simulink library "HANcoder_Linux_Target"  (R2018b)
settings: Solver=ode45  StartTime=0.0  StopTime=10.0  RelTol=1e-3  EnableMultiTasking=on
settings Model: Creator=HANcoder  LastModifiedBy=rickg
settings Model: ModifiedHistory=|
  | la_obwlf -- Thu Sep 01 12:12:55 2016 -- Version 0.33
  | 
  | 
  | 
  | 
  | 
  | 
  | la_obwlf -- Thu Sep 01 09:23:34 2016 -- Version 0.33
  | changed the version in the Base Sample Time block
  | 
  | 
  | 
  | la_obwlf -- Tue Aug 30 15:48:17 2016 -- Version 0.33
settings DataIOCC: LimitDataPoints=on  SaveFormat=Array  SignalLoggingSaveFormat=ModelDataLogs
settings OptimizationCC: ExpressionDepthLimit=2147483647  LifeSpan=inf
settings DebuggingCC: UnderspecifiedInitializationDetection=Classic  MergeDetectMultiDrivingBlocksExec=none  SolverPrmCheckMsg=warning  FcnCallInpInsideContextMsg=warning  StateNameClashWarn=warning  SFUnexpectedBacktrackingDiag=warning  SFNoUnconditionalDefaultTransitionDiag=warning  SFExecutionAtInitializationDiag=none
settings HardwareCC: ProdBitPerPointer=32  ProdBitPerSizeT=32  ProdBitPerPtrDiffT=32  ProdLargestAtomicFloat=None  ProdIntDivRoundTo=Undefined  ProdEndianess=Unspecified  ProdWordSize=32  ProdHWDeviceType=32-bit Generic
settings ModelReferenceCC: PropagateSignalLabelsOutOfModel=off
settings SFSimCC: SimUseLocalCustomCode=off
settings RTWCC: RTWUseLocalCustomCode=off
settings CodeAppCC: StateflowObjectComments=on
settings GRTTargetCC: TargetLangStandard=C89/C90 (ANSI)  GeneratePreprocessorConditionals=Disable all  CombineOutputUpdateFcns=off  GRTInterface=on
settings ConfigComp: CovMetricSettings=dw  CovHtmlReporting=on  CovSaveCumulativeToWorkspaceVar=on  CovSaveSingleToWorkspaceVar=on  CovExternalEMLEnable=off  CovSFcnEnable=off

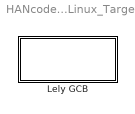
== system HANcoder_Linux_Target ==
  Lely GCB : Subsystem
      mask Display:
      | disp('Lely GCB')
      | patch([80 86 86],[8 14 2],[1 0 0]);patch([88 88 94],[14 2 8],[0 0 0.35]);

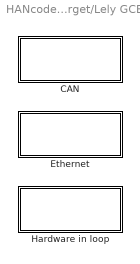
== system HANcoder_Linux_Target/Lely GCB ==
  CAN : Subsystem
      mask Display: fprintf('CAN');patch([85 91 91],[8 14 2],[1 0 0]);patch([93 93 99],[14 2 8],[0 0 0.35]);
  Ethernet : Subsystem
      mask Display: fprintf('Ethernet');patch([85 91 91],[8 14 2],[1 0 0]);patch([93 93 99],[14 2 8],[0 0 0.35]);
  Hardware in loop : Subsystem
      mask Display: fprintf('Hardware in the Loop');patch([85 91 91],[8 14 2],[1 0 0]);patch([93 93 99],[14 2 8],[0 0 0.35]);

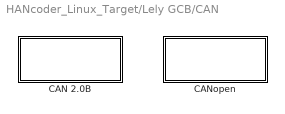
== system HANcoder_Linux_Target/Lely GCB/CAN ==
  CAN 2.0B : Subsystem
      mask Display: fprintf('CAN 2.0B');patch([85 91 91],[8 14 2],[1 0 0]);patch([93 93 99],[14 2 8],[0 0 0.35]);
  CANopen : Subsystem
      mask Display: fprintf('CANopen');patch([85 91 91],[8 14 2],[1 0 0]);patch([93 93 99],[14 2 8],[0 0 0.35]);

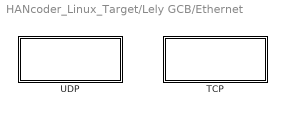
== system HANcoder_Linux_Target/Lely GCB/Ethernet ==
  TCP : Subsystem
      mask Display: fprintf('TCP');patch([85 91 91],[8 14 2],[1 0 0]);patch([93 93 99],[14 2 8],[0 0 0.35]);
  UDP : Subsystem
      mask Display: fprintf('UDP');patch([85 91 91],[8 14 2],[1 0 0]);patch([93 93 99],[14 2 8],[0 0 0.35]);

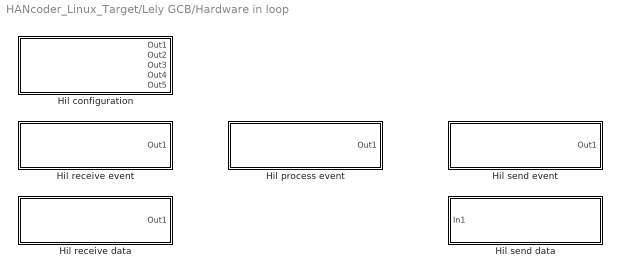
== system HANcoder_Linux_Target/Lely GCB/Hardware in loop ==
  Hil configuration : Subsystem  Tag=HANcoder_TARGET_STM32_Olimexino  mask{tsamp=1, hilSpeed=100, hilConf=HiL Master + 4 Slaves, hilTimeSlot=4, ip1=10, ip2=4, ip3=1, ip4=Automatically assigned by HiL}
      mask prompts: tsamp "Sample time"; hilSpeed "HiL cycle time (ms)"; hilConf "HiL configuration"; hilTimeSlot "Time slot to start"; ip1 "Adress 1"; ip2 "Adress 2"; ip3 "Adress 3"; ip4 "Adress 4"
      mask init:
      | configurationInfoString = sfcn_hil_mcb(hilConf,hilSpeed,hilTimeSlot,ip1,ip2,ip3)
      mask TypeOptions hilConf: HiL Master | HiL Master + 1 Slave | HiL Master + 2 Slaves | HiL Master + 3 Slaves | HiL Master + 4 Slaves
      mask TypeOptions hilTimeSlot: 4 | 5 | 6 | 7 | 8 | 9 | 10
      mask DialogControl Container4 Prompt: HiL parameters
      mask DialogControl Container3 Prompt: IO module IP range
      mask Display:
      | %%port_label('output', 1, 'Time slot');
      | %%port_label('output', 2, 'Sample counter');
      | %%port_label('output', 3, 'Samples lost');
      | %%port_label('output', 4, 'Plant model time');
      | fprintf('Hil Linux GCB\n Hil cycle speed: %d ms\n Setup: %s',hilSpeed,configurationInfoString);
      | patch([135 141 141],[8 14 2],[1 0 0]);patch([143 143 149],[14 2 8],[0 0 0.35]);
  Hil process event : Subsystem  Tag=HANcoder_TARGET_STM32_E407
      mask init:
      | sfcn_hil_process_irq_mcb();
      settings: MoveFcn=%%drawLogos
      mask Display: fprintf('Hil process\nInitiate process event');patch([135 141 141],[8 14 2],[1 0 0]);patch([143 143 149],[14 2 8],[0 0 0.35]);
  Hil receive data : Subsystem  Tag=HANcoder_TARGET_STM32_Olimexino  mask{ioModule=HiL Master, channel=1, datatype=int8}
      mask prompts: ioModule "Smart IO module"; channel "Signal channel"
      mask init:
      | [ioModuleinfoStr] = sfcn_hil_receive_data_mcb(ioModule, channel, datatype);
      mask TypeOptions ioModule: HiL Master | HiL Slave 1 | HiL Slave 2 | HiL Slave 3 | HiL Slave 4
      mask TypeOptions channel: 1 | 2 | 3 | 4 | 5 | 6 | 7 | 8 | 9 | 10 | 11 | 12 | 13 | 14 | 15 | 16 | 17 | 18 | 19 | 20
      mask TypeOptions datatype: int8 | uint8 | int16 | uint16 | int32 | uint32 | boolean
      mask Display: fprintf('Hil get data from\n%s\nChannel %d',ioModuleinfoStr, channel);patch([135 141 141],[8 14 2],[1 0 0]);patch([143 143 149],[14 2 8],[0 0 0.35]);
  Hil receive event : Subsystem  Tag=HANcoder_TARGET_STM32_E407
      mask init:
      | sfcn_hil_receive_irq_mcb();
      settings: MoveFcn=%%drawLogos
      mask Display: fprintf('Hil receive\nData received event');patch([135 141 141],[8 14 2],[1 0 0]);patch([143 143 149],[14 2 8],[0 0 0.35]);
  Hil send data : Subsystem  Tag=HANcoder_TARGET_STM32_Olimexino  mask{ioModule=HiL Master, channel=1, datatype=int8}
      mask prompts: ioModule "Smart IO module"; channel "Signal channel"
      mask init:
      | [ioModuleinfoStr] = sfcn_hil_send_data_mcb(ioModule, channel, datatype);
      mask TypeOptions ioModule: HiL Master | HiL Slave 1 | HiL Slave 2 | HiL Slave 3 | HiL Slave 4
      mask TypeOptions channel: 1 | 2 | 3 | 4 | 5 | 6 | 7 | 8 | 9 | 10 | 11 | 12 | 13 | 14 | 15 | 16 | 17 | 18 | 19 | 20
      mask TypeOptions datatype: int8 | uint8 | int16 | uint16 | int32 | uint32 | boolean
      mask Display: fprintf('Hil send data to\n%s\nChannel %d',ioModuleinfoStr, channel);patch([135 141 141],[8 14 2],[1 0 0]);patch([143 143 149],[14 2 8],[0 0 0.35]);
  Hil send event : Subsystem  Tag=HANcoder_TARGET_STM32_E407
      mask init:
      | sfcn_hil_send_irq_mcb();
      settings: MoveFcn=%%drawLogos
      mask Display: fprintf('Hil send\nInitiate send event');patch([135 141 141],[8 14 2],[1 0 0]);patch([143 143 149],[14 2 8],[0 0 0.35]);

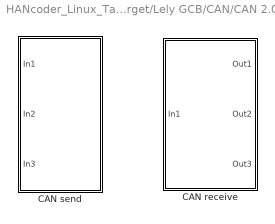
== system HANcoder_Linux_Target/Lely GCB/CAN/CAN 2.0B ==
  CAN receive : Subsystem  Tag=HANcoder_TARGET_STM32_Olimexino  mask(CAN receive){canBus=CAN 1, outputNumber=2, dataType=uint8, byteOrder=off, tsamp=1}
      mask prompts: canBus "CAN channel"; outputNumber "Output ports"; dataType "Output datatype"; byteOrder "Byte order: Checked = MSB first, unchecked = LSB first."; tsamp "Sample time"
      mask help:
      | Function
      | ==========
      | Receive the newest message from the specified CAN channel.
      |
      | Parameters
      | ==========
      | CAN channel:             The CAN channel to send the message on.
      | Output ports:             The amount of output ports
      | Output datatype:       The datatype of the output ports
      | Byte order:                 Select MSB or LSB first
      | Sample time:              -1 or divisible by base sample time [seconds]
      |
      | Input
      | ==========
      | Port 1:                       CAN ID(uint32) in hexadecimal ie: hex2dec('0a')
      |
      | Output
      | ==========
      | Port 1:                       Checks for new message(int8)
      | Port 2..9                     Message data
      mask init:
      | sfcn_can_receive_mcb(canBus, outputNumber, dataType, byteOrder)
      mask Help: web('sfcn_can_receive.html');
      mask TypeOptions canBus: CAN 1
      mask TypeOptions dataType: int8 | uint8 | int16 | uint16 | int32 | uint32 | boolean
      mask Display:
      | fprintf('Receive on\nCAN %x', canBus);
      | port_label('output', 1, 'new')
      | port_label('input', 1, 'ID');patch([75 81 81],[8 14 2],[1 0 0]);patch([83 83 89],[14 2 8],[0 0 0.35]);
  CAN send : Subsystem  Tag=HANcoder_TARGET_STM32_Olimexino  mask(CAN send){canBus=CAN0, frameType=Standard (11 bit), inputNumber=2, dataType=uint8, byteOrder=on, tsamp=0.5}
      mask prompts: canBus "CAN channel"; frameType "Identifier type"; inputNumber "Input ports"; dataType "Input datatype"; byteOrder "Byte order: Checked = MSB first, unchecked = LSB first."; tsamp "Sample time"
      mask help:
      | Function
      | ==========
      | Send a message on the CAN channel.
      |
      | Parameters
      | ==========
      | CAN channel:           The CAN channel to send the message on.
      | Identifier type:         normal or extended ID's
      | Input ports:              The amount of input ports
      | Input datatype:        The datatype of the input ports
      | Byte order:               Select MSB or LSB first
      | Sample time:            -1 or divisible by base sample time [seconds]
      |
      | Input
      | ==========
      | Port 1:                   CAN ID(uint32) in hexadecimal ie: hex2dec('0a')
      | Port 2..9                CAN message data
      mask init:
      | sfcn_can_send_mcb(canBus, frameType, inputNumber, dataType, byteOrder)
      mask Help: web('sfcn_can_send.html');
      mask TypeOptions canBus: CAN0 | CAN1
      mask TypeOptions frameType: Standard (11 bit) | Extended (29 bit)
      mask TypeOptions dataType: int8 | uint8 | int16 | uint16 | int32 | uint32 | boolean
      mask Display:
      | fprintf('Send on\nCAN%x', canBus-1);
      | port_label('input', 1, 'ID');patch([65 71 71],[8 14 2],[1 0 0]);patch([73 73 79],[14 2 8],[0 0 0.35]);

== system HANcoder_Linux_Target/Lely GCB/CAN/CANopen ==

== system HANcoder_Linux_Target/Lely GCB/Ethernet/TCP ==

== system HANcoder_Linux_Target/Lely GCB/Ethernet/UDP ==
  UDP Client Send : Subsystem  Tag=HANcoder_TARGET_STM32_Olimexino  mask(UDP Client Send){ip1=10, ip2=4, ip3=1, ip4=10, port=2000, inputNumber=1, dataType=int8, byteOrder=on, tsamp=-1}
      mask prompts: ip1 "IP address 1"; ip2 "IP address 2"; ip3 "IP address 3"; ip4 "IP address 4"; port "Port2"; inputNumber "Input ports"; dataType "Input datatype"; byteOrder "Byte order: Checked = MSB first, unchecked = LSB first."; tsamp "Sample time"
      mask help:
      | Function
      | ========
      | Sends a data packet to the UDP server with the specified IP address on
      | the specified port.
      |
      | Parameters
      | ==========
      | IP address 1:   First quad of the UDP server's IP address.
      | IP address 2:   Second quad of the UDP server's IP address.
      | IP address 3:   Third quad of the UDP server's IP address.
      | IP address 4:   Fourth quad of the UDP server's IP address.
      | Port:           Port to send the data packet on.
      | Input ports:    The amount of input ports.
      | Input datatype: The datatype of the input ports.
      | Byte order:     Select MSB or LSB first.
      | Sample time:    -1 or divisible by base sample time [seconds].
      |
      | Input
      | =====
      | Port 1..32      UDP packet data.
      mask init:
      | sfcn_udp_client_send_mcb(ip1,ip2,ip3,ip4,port,inputNumber,dataType,byteOrder);
      mask Help: web('sfcn_udp_client_send.html');
      mask TypeOptions inputNumber: 1 | 2 | 3 | 4 | 5 | 6 | 7 | 8 | 9 | 10 | 11 | 12 | 13 | 14 | 15 | 16 | 17 | 18 | 19 | 20 | 21 | 22 | 23 | 24 | 25 | 26 | 27 | 28 | 29 | 30 | 31 | 32
      mask TypeOptions dataType: int8 | uint8 | int16 | uint16 | int32 | uint32 | boolean
      mask Display:
      | fprintf('UDP Client Send');patch([125 131 131],[8 14 2],[1 0 0]);patch([133 133 139],[14 2 8],[0 0 0.35]);
      | %fprintf('UDP Client Send\n\nport: %d\nip: %d.%d.%d.%d', port, ip1, ip2, ip3, ip4);patch([125 131 131],[8 14 2],[1 0 0]);patch([133 133 139],[14 2 8],[0 0 0.35]);
  UDP Server Receive : Subsystem  Tag=HANcoder_TARGET_STM32_Olimexino  mask(UDP Server Receive){outputNumber=10, dataType=int8, byteOrder=on, startIdx=1, tsamp=-1}
      mask prompts: outputNumber "Output ports"; dataType "Output datatype"; byteOrder "Byte order: Checked = MSB first, unchecked = LSB first."; startIdx "Start index"; tsamp "Sample time"
      mask help:
      | Function
      | ========
      | Reads data from the UDP server's internal receive buffer.
      |
      | Parameters
      | ==========
      | Output ports:    The amount of output ports.
      | Output datatype: The datatype of the output ports.
      | Byte order:      Select MSB or LSB first.
      | Start index:     Start index in the server's buffer to start reading from.
      | Sample time:     -1 or divisible by base sample time [seconds].
      |
      | Output
      | ======
      | Port 1..32       UDP received packet data.
      mask init:
      | sfcn_udp_server_receive_mcb(outputNumber, dataType, byteOrder, startIdx);
      mask Help: web('sfcn_udp_client_send.html');
      mask TypeOptions outputNumber: 1 | 2 | 3 | 4 | 5 | 6 | 7 | 8 | 9 | 10 | 11 | 12 | 13 | 14 | 15 | 16 | 17 | 18 | 19 | 20 | 21 | 22 | 23 | 24 | 25 | 26 | 27 | 28 | 29 | 30 | 31 | 32
      mask TypeOptions dataType: int8 | uint8 | int16 | uint16 | int32 | uint32 | boolean
      mask TypeOptions startIdx: 1 | 2 | 3 | 4 | 5 | 6 | 7 | 8 | 9 | 10 | 11 | 12 | 13 | 14 | 15 | 16 | 17 | 18 | 19 | 20 | 21 | 22 | 23 | 24 | 25 | 26 | 27 | 28 | 29 | 30 | 31 | 32
      mask Display: fprintf('UDP Server Receive');patch([130 136 136],[8 14 2],[1 0 0]);patch([138 138 144],[14 2 8],[0 0 0.35]);

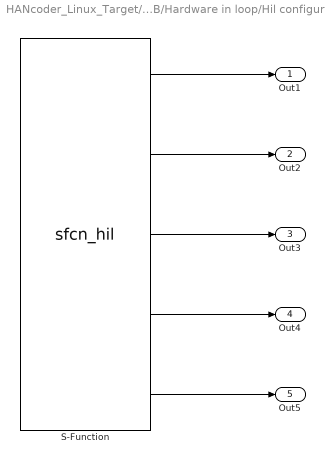
== system HANcoder_Linux_Target/Lely GCB/Hardware in loop/Hil configuration ==
  S-Function : M-S-Function  FunctionName=sfcn_hil  Parameters=tsamp, hilConf,hilSpeed,hilTimeSlot,ip1,ip2,ip3
  Out1 : Outport
  Out2 : Outport  Port=2
  Out3 : Outport  Port=3
  Out4 : Outport  Port=4
  Out5 : Outport  Port=5
  wires:
  S-Function/1 -> Out1/1
  S-Function/2 -> Out2/1
  S-Function/3 -> Out3/1
  S-Function/4 -> Out4/1
  S-Function/5 -> Out5/1

== system HANcoder_Linux_Target/Lely GCB/Hardware in loop/Hil process event ==
  S-Function : S-Function  FunctionName=sfcn_hil_process_irq  SFunctionDeploymentMode=off  EnableBusSupport=off
  Out1 : Outport
  wires:
  S-Function/1 -> Out1/1

== system HANcoder_Linux_Target/Lely GCB/Hardware in loop/Hil receive data ==
  S-Function : M-S-Function  FunctionName=sfcn_hil_receive_data  Parameters=ioModule, channel, datatype
  Out1 : Outport
  wires:
  S-Function/1 -> Out1/1

== system HANcoder_Linux_Target/Lely GCB/Hardware in loop/Hil receive event ==
  S-Function : S-Function  FunctionName=sfcn_hil_receive_irq  SFunctionDeploymentMode=off  EnableBusSupport=off
  Out1 : Outport
  wires:
  S-Function/1 -> Out1/1

== system HANcoder_Linux_Target/Lely GCB/Hardware in loop/Hil send data ==
  In1 : Inport
  S-Function : M-S-Function  FunctionName=sfcn_hil_send_data  Parameters=ioModule, channel, datatype
  wires:
  In1/1 -> S-Function/1

== system HANcoder_Linux_Target/Lely GCB/Hardware in loop/Hil send event ==
  S-Function : S-Function  FunctionName=sfcn_hil_send_irq  SFunctionDeploymentMode=off  EnableBusSupport=off
  Out1 : Outport
  wires:
  S-Function/1 -> Out1/1

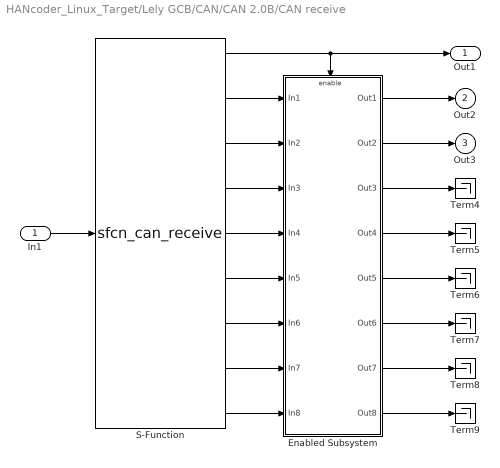
== system HANcoder_Linux_Target/Lely GCB/CAN/CAN 2.0B/CAN receive ==
  In1 : Inport
  Enabled Subsystem : Subsystem  TreatAsAtomicUnit=on
  S-Function : M-S-Function  FunctionName=sfcn_can_receive  Parameters=tsamp, canBus, outputNumber, dataType, byteOrder
  Term{4..9} (6 alike) : Terminator
  Out1 : Outport
  Out2 : Outport  Port=2
  Out3 : Outport  Port=3
  wires:
  Enabled Subsystem/8(Out8) -> Term9/1
  Enabled Subsystem/7(Out7) -> Term8/1
  Enabled Subsystem/6(Out6) -> Term7/1
  Enabled Subsystem/5(Out5) -> Term6/1
  Enabled Subsystem/4(Out4) -> Term5/1
  Enabled Subsystem/3(Out3) -> Term4/1
  Enabled Subsystem/2(Out2) -> Out3/1
  Enabled Subsystem/1(Out1) -> Out2/1
  S-Function/7 -> Enabled Subsystem/6(In6)
  S-Function/8 -> Enabled Subsystem/7(In7)
  S-Function/4 -> Enabled Subsystem/3(In3)
  S-Function/3 -> Enabled Subsystem/2(In2)
  S-Function/2 -> Enabled Subsystem/1(In1)
  S-Function/9 -> Enabled Subsystem/8(In8)
  S-Function/5 -> Enabled Subsystem/4(In4)
  S-Function/6 -> Enabled Subsystem/5(In5)
  S-Function/1 -> Out1/1, Enabled Subsystem/Enable
  In1/1 -> S-Function/1

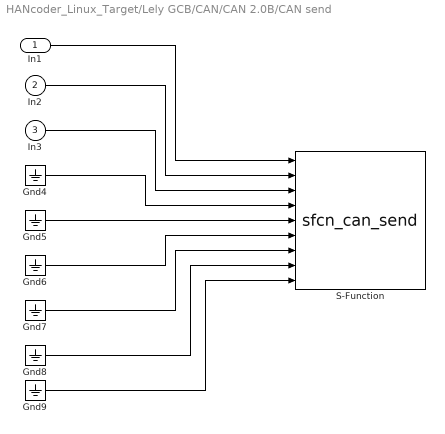
== system HANcoder_Linux_Target/Lely GCB/CAN/CAN 2.0B/CAN send ==
  In1 : Inport
  In2 : Inport  Port=2
  In3 : Inport  Port=3
  Gnd{4..9} (6 alike) : Ground
  S-Function : M-S-Function  FunctionName=sfcn_can_send  Parameters=tsamp, canBus, frameType, inputNumber, dataType, byteOrder
  wires:
  Gnd9/1 -> S-Function/9
  Gnd8/1 -> S-Function/8
  Gnd7/1 -> S-Function/7
  Gnd6/1 -> S-Function/6
  Gnd5/1 -> S-Function/5
  Gnd4/1 -> S-Function/4
  In3/1 -> S-Function/3
  In2/1 -> S-Function/2
  In1/1 -> S-Function/1

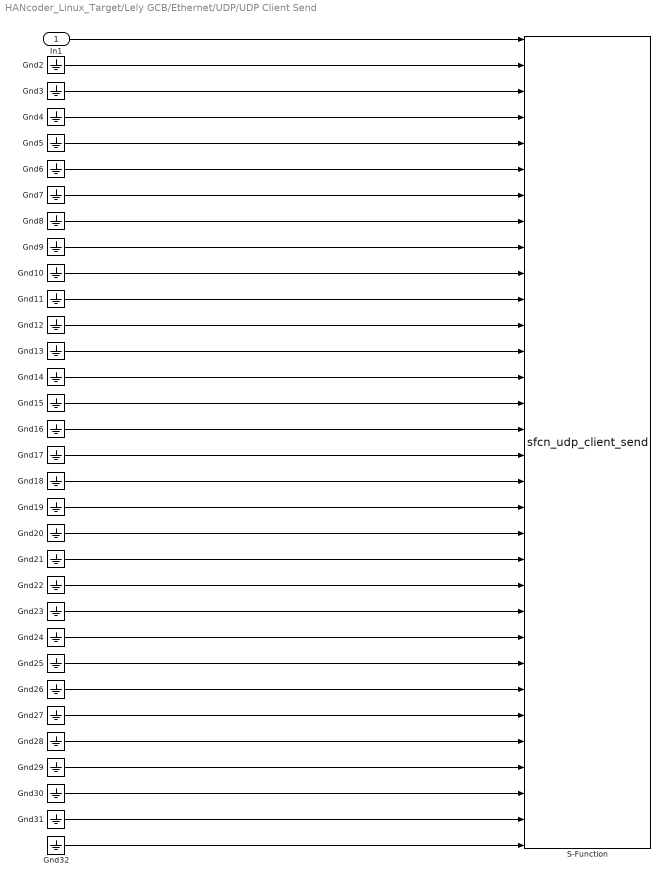
== system HANcoder_Linux_Target/Lely GCB/Ethernet/UDP/UDP Client Send ==
  In1 : Inport
  Gnd{2..32} (31 alike) : Ground
  S-Function : M-S-Function  FunctionName=sfcn_udp_client_send  Parameters=tsamp, dataType
  wires:
  Gnd9/1 -> S-Function/9
  Gnd8/1 -> S-Function/8
  Gnd7/1 -> S-Function/7
  Gnd6/1 -> S-Function/6
  Gnd5/1 -> S-Function/5
  Gnd4/1 -> S-Function/4
  Gnd3/1 -> S-Function/3
  Gnd2/1 -> S-Function/2
  In1/1 -> S-Function/1
  Gnd13/1 -> S-Function/13
  Gnd14/1 -> S-Function/14
  Gnd15/1 -> S-Function/15
  Gnd16/1 -> S-Function/16
  Gnd12/1 -> S-Function/12
  Gnd11/1 -> S-Function/11
  Gnd10/1 -> S-Function/10
  Gnd18/1 -> S-Function/18
  Gnd20/1 -> S-Function/20
  Gnd22/1 -> S-Function/22
  Gnd17/1 -> S-Function/17
  Gnd19/1 -> S-Function/19
  Gnd23/1 -> S-Function/23
  Gnd28/1 -> S-Function/28
  Gnd29/1 -> S-Function/29
  Gnd27/1 -> S-Function/27
  Gnd26/1 -> S-Function/26
  Gnd25/1 -> S-Function/25
  Gnd21/1 -> S-Function/21
  Gnd30/1 -> S-Function/30
  Gnd31/1 -> S-Function/31
  Gnd24/1 -> S-Function/24
  Gnd32/1 -> S-Function/32

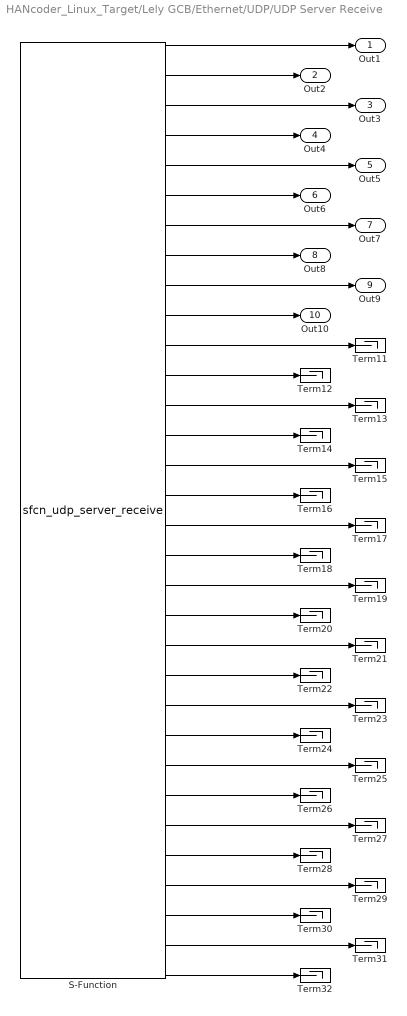
== system HANcoder_Linux_Target/Lely GCB/Ethernet/UDP/UDP Server Receive ==
  S-Function : M-S-Function  FunctionName=sfcn_udp_server_receive  Parameters=tsamp, dataType
  Term{11..32} (22 alike) : Terminator
  Out1 : Outport
  Out2 : Outport  Port=2
  Out3 : Outport  Port=3
  Out4 : Outport  Port=4
  Out5 : Outport  Port=5
  Out6 : Outport  Port=6
  Out7 : Outport  Port=7
  Out8 : Outport  Port=8
  Out9 : Outport  Port=9
  Out10 : Outport  Port=10
  wires:
  S-Function/32 -> Term32/1
  S-Function/31 -> Term31/1
  S-Function/30 -> Term30/1
  S-Function/29 -> Term29/1
  S-Function/28 -> Term28/1
  S-Function/27 -> Term27/1
  S-Function/26 -> Term26/1
  S-Function/25 -> Term25/1
  S-Function/24 -> Term24/1
  S-Function/23 -> Term23/1
  S-Function/22 -> Term22/1
  S-Function/21 -> Term21/1
  S-Function/20 -> Term20/1
  S-Function/19 -> Term19/1
  S-Function/18 -> Term18/1
  S-Function/17 -> Term17/1
  S-Function/16 -> Term16/1
  S-Function/15 -> Term15/1
  S-Function/14 -> Term14/1
  S-Function/13 -> Term13/1
  S-Function/1 -> Out1/1
  S-Function/2 -> Out2/1
  S-Function/3 -> Out3/1
  S-Function/4 -> Out4/1
  S-Function/5 -> Out5/1
  S-Function/6 -> Out6/1
  S-Function/7 -> Out7/1
  S-Function/8 -> Out8/1
  S-Function/9 -> Out9/1
  S-Function/10 -> Out10/1
  S-Function/12 -> Term12/1
  S-Function/11 -> Term11/1

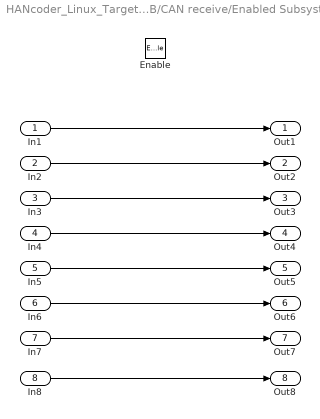
== system HANcoder_Linux_Target/Lely GCB/CAN/CAN 2.0B/CAN receive/Enabled Subsystem ==
  In1 : Inport
  In2 : Inport  Port=2
  In3 : Inport  Port=3
  In4 : Inport  Port=4
  In5 : Inport  Port=5
  In6 : Inport  Port=6
  In7 : Inport  Port=7
  In8 : Inport  Port=8
  Enable : EnablePort
  Out1 : Outport
  Out2 : Outport  Port=2
  Out3 : Outport  Port=3
  Out4 : Outport  Port=4
  Out5 : Outport  Port=5
  Out6 : Outport  Port=6
  Out7 : Outport  Port=7
  Out8 : Outport  Port=8
  wires:
  In8/1 -> Out8/1
  In7/1 -> Out7/1
  In6/1 -> Out6/1
  In5/1 -> Out5/1
  In4/1 -> Out4/1
  In3/1 -> Out3/1
  In2/1 -> Out2/1
  In1/1 -> Out1/1
